simulink model "VehicleDynamics3D_controller"  (R2017a)
settings: Solver=ode45  StartTime=0.0  StopTime=stoptime  FixedStep=.001  MaxStep=maxStep  RelTol=relTol  AbsTol=absTol  EnableMultiTasking=on
PreLoadFcn:
  | VehicleDynamicsInitialization
model workspace: external: MATLAB File sm_suspension_templates_params.m (data not in the file)
values from neighbouring files (symbols this model uses):
  D = 0.1341    [Run_VehicleDynamics3D.m]
  Dt = 0.65979    [Run_VehicleDynamics3D.m]
  I = 0.55564    [Run_VehicleDynamics3D.m]
  It = 0.7671    [Run_VehicleDynamics3D.m]
  latv_setpoint = -12.28    [Run_VehicleDynamics3D.m]
  max_speed = 80    [Run_VehicleDynamics3D.m]
  P = 1.2095    [Run_VehicleDynamics3D.m]
  Pt = 2.1389    [Run_VehicleDynamics3D.m]
  ste_gain = 1    [Run_VehicleDynamics3D.m]
  steering_step = -30    [Run_VehicleDynamics3D.m]
  switch_speed_control = 3.28    [Run_VehicleDynamics3D.m]
  switch_steering = 100    [Run_VehicleDynamics3D.m]
  switch_steering_control = 3.58    [Run_VehicleDynamics3D.m]
  switch_throttle = 3.28    [Run_VehicleDynamics3D.m]
  thl_gain = 1    [Run_VehicleDynamics3D.m]
undefined symbols (not defined in the file or in its folder): dwb, Floor, followerCameraX, followerCameraZ, frontCameraX, frontCameraZ, isoCameraAimX, isoCameraX, isoCameraY, isoCameraZ, Load, maxSteeringDisplacement, minSteeringDisplacement, SetPaceSampleTime, wheel, wheelbase, X, Y, Z
libraries: sm_lib x199, sm_suspension_templates_lib x34, nesl_utility x20, simulink x8, fl_lib x7, Contact_Forces_Lib x4, aerolibanimutils x1
(part 1 of 7)
CloseFcn:
  | clear simlog_sm_suspension_templates
Description:
  | Independent Suspension System Templates
  | 
  | Copyright 2016-2017 The MathWorks, Inc.
settings Model: Creator=MathWorks  LastModifiedBy=regab
settings SolverCC: ZeroCrossAlgorithm=Adaptive
settings DataIOCC: SaveFormat=Array  SaveOutput=off  ReturnWorkspaceOutputs=on  ReturnWorkspaceOutputsName=FrameCopy_spidata
settings OptimizationCC: ExpressionDepthLimit=2147483647  LifeSpan=inf
settings DebuggingCC: UnderspecifiedInitializationDetection=Classic  MergeDetectMultiDrivingBlocksExec=none  MaskedZcDiagnostic=none  IgnoredZcDiagnostic=none  AllowSymbolicDim=off  StateNameClashWarn=warning  SFUnexpectedBacktrackingDiag=warning  SFNoUnconditionalDefaultTransitionDiag=warning  SFExecutionAtInitializationDiag=none
settings HardwareCC: ProdBitPerPointer=32  ProdBitPerSizeT=32  ProdBitPerPtrDiffT=32  ProdLargestAtomicFloat=None  ProdIntDivRoundTo=Undefined  ProdEndianess=Unspecified  ProdWordSize=32  ProdHWDeviceType=32-bit Generic
settings ModelReferenceCC: PropagateSignalLabelsOutOfModel=off
settings SFSimCC: SimBuildMode=sf_make
settings GRTTargetCC: TargetLangStandard=C89/C90 (ANSI)  GeneratePreprocessorConditionals=Disable all
settings ConfigComp: CovScope=ReferencedModels  CovIncludeTopModel=off  CovMetricSettings=dw  CovHtmlReporting=on  CovSaveCumulativeToWorkspaceVar=on  CovSaveSingleToWorkspaceVar=on  CovExternalEMLEnable=off  CovSFcnEnable=off
settings SimscapeCC: SimscapeLogSimulationStatistics=on  SimscapeLogLimitData=off  SimscapeLogDataHistory=10000
settings ConfigurationSet: Description=SimMechanics 2G
settings DiagnosticsConfigSet: SimMechanicsUnconnectedFramePorts=none  SimMechanicsRigidlyBoundBlock=none  SimMechanicsUnsatisfiedHighPriorityTargets=none
settings ExplorerConfigSet: InternalSimMechanicsExplorerSettings="<ExplorerConfiguration><canonicalview>default</canonicalview><AnimationSetting><BasePlaybackSpeed>1.0</BasePlaybackSpeed><PlaybackSpeedFactor>1.0</PlaybackSpeedFactor></AnimationSetting><TilePanel><TileInfo><Tiles Columns=\"2\" Count=\"3\" Rows=\"2\"><Column Left=\"2\" Weight=\"0.4529\"/><Column Left=\"381\" Weight=\"0.5471\"/><Column Left=\"837\"/><Row Top=\"2\" Weight=\"0.5729\"/><Row Top=\"598\" Weight=\"0.4271\"/><Row Top=\"1044\"/><Tile Height=\"2\" Width=\"1\" X=\"0\" Y=\"0\"/><Tile Height=\"1\" Width=\"1\" X=\"1\" Y=\"0\"/><Tile Height=\"1\" Width=\"1\" X=\"1\" Y=\"1\"/></Tiles></TileInfo><SceneInfo><SceneViewer><BGColor><R>0.60000002384185791</R><G>0.60000002384185791</G><B>0.60000002384185791</B></BGColor><Camera><DoPerspective>on</DoPerspective><Position><X>-1.1537063873740901e-15</X><Y>-7.5000000000000018</Y><Z>3.2999999999999994</Z></Position><Center><X>6.6613381477509392e-16</X><Y>1.1102230246251565e-16</Y><Z>0.29999999999999993</Z></Center><Up><X>-5.1501888403816389e-17</X><Y>-7.1161584930853499e-17</Y><Z>1</Z></Up><ViewLimDist>1</ViewLimDist><YLim>0.46630765815499858</YLim><XLim>0.16702210408262291</XLim></Camera></SceneViewer><SceneViewer><BGColor><R>0.60000002384185791</R><G>0.60000002384185791</G><B>0.60000002384185791</B></BGColor><Camera><DoPerspective>on</DoPerspective><Position><X>3.5000000000000018</X><Y>3.0999999999999996</Y><Z>1.8000000000000003</Z></Position><Center><X>4.9960036108132044e-16</X><Y>-0.75000000000000011</Y><Z>0.29999999999999988</Z></Center><Up><X>0</X><Y>0</Y><Z>1</Z></Up><ViewLimDist>1</ViewLimDist><YLim>0.46630765815499858</YLim><XLim>0.35509288448941123</XLim></Camera></SceneViewer><SceneViewer><BGColor><R>0.60000002384185791</R><G>0.60000002384185791</G><B>0.60000002384185791</B></BGColor><Camera><DoPerspective>on</DoPerspective><Position><X>1.036686212452563e-15</X><Y>1.7500000000000004</Y><Z>0.65000000000000002</Z></Position><Center><X>6.6613381477509392e-16</X><Y>1.1102230246251565e-16</Y><Z>0.29999999999999993</Z></Center><Up><X>-5.1501888403816389e-17</X><Y>-7.1161584930853499e-17</Y><Z>1</Z></Up><ViewLimDist>1</ViewLimDist><YLim>0.46630765815499858</YLim><XLim>0.47697831394801909</XLim></Camera></SceneViewer></SceneInfo></TilePanel><MechEditorPanel><Cameras><Camera><Id>Camera1</Id><Value><Name>Follower Camera</Name><NativeCamera><PositionTrackingFeature>Cameras.Follower_Camera_Transform.F</PositionTrackingFeature><CenterTrackingFeature>Cameras.Follower_Camera_Transform.B</CenterTrackingFeature><UpVectorTrackingFeature>Cameras.Follower_Camera_Transform.B</UpVectorTrackingFeature><CenterTrackingOrigin>on</CenterTrackingOrigin><UpVectorTrackingDirection>+Z</UpVectorTrackingDirection></NativeCamera></Value></Camera><Camera><Id>Camera2</Id><Value><Name>Isometric Camera</Name><NativeCamera><PositionTrackingFeature>Cameras.Isometric_Camera_Transform.F</PositionTrackingFeature><CenterTrackingFeature>Cameras.Isometric_Camera_Aim.F</CenterTrackingFeature><UpVectorTrackingFeature>Floor_And_Grid.World_Frame.W</UpVectorTrackingFeature><CenterTrackingOrigin>on</CenterTrackingOrigin><UpVectorTrackingDirection>+Z</UpVectorTrackingDirection></NativeCamera></Value></Camera><Camera><Id>Camera3</Id><Value><Name>Front Camera</Name><NativeCamera><PositionTrackingFeature>Cameras.Front_Camera_Transform.F</PositionTrackingFeature><CenterTrackingFeature>Cameras.Front_Camera_Transform.B</CenterTrackingFeature><UpVectorTrackingFeature>Cameras.Front_Camera_Transform.B</UpVectorTrackingFeature><CenterTrackingOrigin>on</CenterTrackingOrigin><UpVectorTrackingDirection>+Z</UpVectorTrackingDirection></NativeCamera></Value></Camera></Cameras><GfxPanelCameraMap><MapElement CameraMLId=\"Camera1\" GfxPanelIndex=\"0\"/><MapElement CameraMLId=\"Camera2\" GfxPanelIndex=\"1\"/><MapElement CameraMLId=\"Camera3\" GfxPanelIndex=\"2\"/></GfxPanelCameraMap><VideoCreator><PlaybackSpeedRatio>1.0</PlaybackSpeedRatio><FrameRate>30</FrameRate><VideoFormat>Motion JPEG AVI</VideoFormat><FrameSize>auto</FrameSize></VideoCreator></MechEditorPanel></ExplorerConfiguration>"

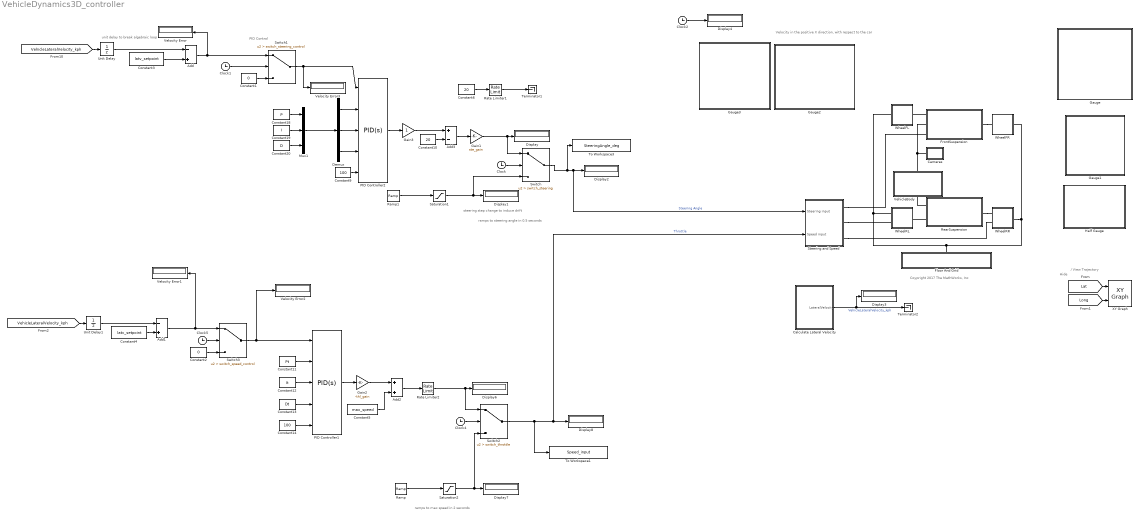
== system VehicleDynamics3D_controller ==
  note: Velocity in the positive X direction, with respect to the car
  note: Hide
  note: / View Trajectory
  note: Coypright 2017 The MathWorks, Inc
  note: ramps to max speed in 2 seconds
  note: unit delay to break algebraic loop
  note: steering step change to induce drift
  note: PID Control
  note: ramps to steering angle in 0.5 seconds
  Add : Sum  Inputs=-+
  Add1 : Sum  Inputs=-+
  Add2 : Sum
  Add3 : Sum  Inputs=+-
  Calculate Lateral Velocity : Subsystem
  Cameras : Subsystem
      mask Display: image('CameraPic.png');
  Clock{,1..2,4..5} (5 alike) : Clock
      Clock settings: Decimation=7
      Clock2 settings: Decimation=7
      Clock4 settings: Decimation=7
  Constant1 : Constant  Value=0
  Constant10 : Constant  Value=20
  Constant11 : Constant  Value=Pt  VectorParams1D=off
  Constant12 : Constant  Value=It
  Constant13 : Constant  Value=Dt
  Constant14 : Constant  Value=100
  Constant18 : Constant  Value=P
  Constant19 : Constant  Value=I
  Constant2 : Constant  Value=0
  Constant20 : Constant  Value=D
  Constant3 : Constant  Value=latv_setpoint
  Constant4 : Constant  Value=latv_setpoint
  Constant5 : Constant  Value=max_speed
  Constant6 : Constant  Value=20
  Constant9 : Constant  Value=100
  Demux : Demux  Outputs=3
  Display{,1..4,6..8} (8 alike) : Display
  Floor And Grid : Subsystem
      mask Display: image('Floor.png');
  FrontSuspension : Subsystem  VariantControl=DoubleWishbone
      mask Display:
      | image(imread(fullfile(matlabroot,...
      |     'toolbox','physmod','sm','smdemos',...
      |     'suspension_templates','images','sm_isuspension_dwishbone.png')));
  Gain1 : Gain  Gain=ste_gain
  Gain2 : Gain  Gain=-thl_gain
  Gain3 : Gain
  Gauge : Subsystem  DialogController=hmiCreateDDGDialog  IsWebBlock=on  mask(MWDashboardBlock){webBlockId=e0acaf17-1707-462e-bd3e-ad1907f2a35e, webBlockType=circulargauge, ShowInLibBrowser=on, ShowInitialText=on, HMISrcModelName=VehicleDynamics3D_controller}
      mask prompts: webBlockId "WebBlock Id"; webBlockType "WebBlock Type"; HMISrcModelName "Source Model"
      mask help: SimulinkHMI:dialogs:CircularGaugeDialogDesc
      mask Help: helpview([docroot '/mapfiles/simulink.map'], 'hmi_gauge')
      mask Display:
      | if strcmp(get_param(bdroot(gcb),'BlockDiagramType'), 'library')
      |     image([(matlabroot) '/toolbox/simulink/hmi/icons/CircularGauge.png']);
      | end
  Gauge1 : Subsystem  DialogController=hmiCreateDDGDialog  IsWebBlock=on  mask(MWDashboardBlock){webBlockId=a4d7a6c9-5cb1-4197-bb1e-6d17cd857777, webBlockType=circulargauge, ShowInLibBrowser=on, ShowInitialText=on, HMISrcModelName=VehicleDynamics3D_controller}
      mask prompts: webBlockId "WebBlock Id"; webBlockType "WebBlock Type"; HMISrcModelName "Source Model"
      mask help: SimulinkHMI:dialogs:CircularGaugeDialogDesc
      mask Help: helpview([docroot '/mapfiles/simulink.map'], 'hmi_gauge')
      mask Display:
      | if strcmp(get_param(bdroot(gcb),'BlockDiagramType'), 'library')
      |     image([(matlabroot) '/toolbox/simulink/hmi/icons/CircularGauge.png']);
      | end
  Gauge2 : Subsystem  DialogController=hmiCreateDDGDialog  IsWebBlock=on  mask(MWDashboardBlock){webBlockId=9138c855-01fc-4053-99a3-41b98eb70a74, webBlockType=circulargauge, ShowInLibBrowser=on, ShowInitialText=on, HMISrcModelName=VehicleDynamics3D_controller}
      mask prompts: webBlockId "WebBlock Id"; webBlockType "WebBlock Type"; HMISrcModelName "Source Model"
      mask help: SimulinkHMI:dialogs:CircularGaugeDialogDesc
      mask Help: helpview([docroot '/mapfiles/simulink.map'], 'hmi_gauge')
      mask Display:
      | if strcmp(get_param(bdroot(gcb),'BlockDiagramType'), 'library')
      |     image([(matlabroot) '/toolbox/simulink/hmi/icons/CircularGauge.png']);
      | end
  Gauge3 : Subsystem  DialogController=hmiCreateDDGDialog  IsWebBlock=on  mask(MWDashboardBlock){webBlockId=2bdbd2f3-79cc-4c0f-8469-e300a5d3b56d, webBlockType=circulargauge, ShowInLibBrowser=on, ShowInitialText=on, HMISrcModelName=VehicleDynamics3D_controller}
      mask prompts: webBlockId "WebBlock Id"; webBlockType "WebBlock Type"; HMISrcModelName "Source Model"
      mask help: SimulinkHMI:dialogs:CircularGaugeDialogDesc
      mask Help: helpview([docroot '/mapfiles/simulink.map'], 'hmi_gauge')
      mask Display:
      | if strcmp(get_param(bdroot(gcb),'BlockDiagramType'), 'library')
      |     image([(matlabroot) '/toolbox/simulink/hmi/icons/CircularGauge.png']);
      | end
  Half Gauge : Subsystem  DialogController=hmiCreateDDGDialog  IsWebBlock=on  mask(MWDashboardBlock){webBlockId=2bf35224-e477-42b1-a6f6-088c116ad7f4, webBlockType=semicirculargauge, ShowInLibBrowser=on, ShowInitialText=on, HMISrcModelName=VehicleDynamics3D_controller}
      mask prompts: webBlockId "WebBlock Id"; webBlockType "WebBlock Type"; HMISrcModelName "Source Model"
      mask help: SimulinkHMI:dialogs:SemicircularGaugeDialogDesc
      mask Help: helpview([docroot '/mapfiles/simulink.map'], 'hmi_half_gauge')
      mask Display:
      | if strcmp(get_param(bdroot(gcb),'BlockDiagramType'), 'library')
      |     image([(matlabroot) '/toolbox/simulink/hmi/icons/SemicircularGauge.png']);
      | end
  Mux1 : Mux  Inputs=3
  PID Controller1 : simulink/Continuous/PID Controller  Controller=PID  TimeDomain=Continuous-time  SampleTime=-1  IntegratorMethod=Forward Euler  FilterMethod=Forward Euler  Form=Parallel  UseFilter=on  ControllerParametersSource=external  P=.7*5  I=.2*4  D=1.2*3  N=100  InitialConditionSource=internal  InitialConditionForIntegrator=0  InitialConditionForFilter=0  ExternalReset=none  LimitOutput=on  UpperSaturationLimit=60  LowerSaturationLimit=-60  LinearizeAsGain=on  AntiWindupMode=none  Kb=4  TrackingMode=off  Kt=1  PParamMin=[]  PParamMax=[]  IParamMin=[]  IParamMax=[]  DParamMin=[]  DParamMax=[]  NParamMin=[]  NParamMax=[]  KbParamMin=[]  KbParamMax=[]  KtParamMin=[]  KtParamMax=[]  POutMin=[]  POutMax=[]  IOutMin=[]  IOutMax=[]  DOutMin=[]  DOutMax=[]  NOutMin=[]  NOutMax=[]  KbOutMin=[]  KbOutMax=[]  KtOutMin=[]  KtOutMax=[]  IntegratorOutMin=[]  IntegratorOutMax=[]  FilterOutMin=[]  FilterOutMax=[]  SumOutMin=[]  SumOutMax=[]  SumI1OutMin=[]  SumI1OutMax=[]  SumI2OutMin=[]  SumI2OutMax=[]  SumI3OutMin=[]  SumI3OutMax=[]  SumDOutMin=[]  SumDOutMax=[]  SaturationOutMin=[]  SaturationOutMax=[]  IntegratorContinuousStateAttributes=''  IntegratorStateMustResolveToSignalObject=off  IntegratorRTWStateStorageClass=Auto  FilterContinuousStateAttributes=''  FilterStateMustResolveToSignalObject=off  FilterRTWStateStorageClass=Auto  DifferentiatorICPrevScaledInput=0  DifferentiatorOutMin=[]  DifferentiatorOutMax=[]
  PID Controller2 : simulink/Continuous/PID Controller  Controller=PID  TimeDomain=Continuous-time  SampleTime=-1  IntegratorMethod=Forward Euler  FilterMethod=Forward Euler  Form=Parallel  UseFilter=on  ControllerParametersSource=external  P=.7*5  I=.2*4  D=1.2*3  N=100  InitialConditionSource=internal  InitialConditionForIntegrator=0  InitialConditionForFilter=0  ExternalReset=none  LimitOutput=on  UpperSaturationLimit=40  LowerSaturationLimit=-40  LinearizeAsGain=on  AntiWindupMode=none  Kb=1  TrackingMode=off  Kt=1  PParamMin=[]  PParamMax=[]  IParamMin=[]  IParamMax=[]  DParamMin=[]  DParamMax=[]  NParamMin=[]  NParamMax=[]  KbParamMin=[]  KbParamMax=[]  KtParamMin=[]  KtParamMax=[]  POutMin=[]  POutMax=[]  IOutMin=[]  IOutMax=[]  DOutMin=[]  DOutMax=[]  NOutMin=[]  NOutMax=[]  KbOutMin=[]  KbOutMax=[]  KtOutMin=[]  KtOutMax=[]  IntegratorOutMin=[]  IntegratorOutMax=[]  FilterOutMin=[]  FilterOutMax=[]  SumOutMin=[]  SumOutMax=[]  SumI1OutMin=[]  SumI1OutMax=[]  SumI2OutMin=[]  SumI2OutMax=[]  SumI3OutMin=[]  SumI3OutMax=[]  SumDOutMin=[]  SumDOutMax=[]  SaturationOutMin=[]  SaturationOutMax=[]  IntegratorContinuousStateAttributes=''  IntegratorStateMustResolveToSignalObject=off  IntegratorRTWStateStorageClass=Auto  FilterContinuousStateAttributes=''  FilterStateMustResolveToSignalObject=off  FilterRTWStateStorageClass=Auto  DifferentiatorICPrevScaledInput=0  DifferentiatorOutMin=[]  DifferentiatorOutMax=[]
  Ramp : simulink/Sources/Ramp  slope=max_speed/2  start=.75  X0=0
  Ramp1 : simulink/Sources/Ramp  slope=steering_step*2  start=steering_step_t  X0=0
  Rate Limiter1 : RateLimiter  RisingSlewLimit=500  FallingSlewLimit=-500  SampleTimeMode=inherited
  Rate Limiter2 : RateLimiter  RisingSlewLimit=50  FallingSlewLimit=-50  SampleTimeMode=inherited
  RearSuspension : Subsystem  VariantControl=DoubleWishbone
      mask Display:
      | image(imread(fullfile(matlabroot,...
      |     'toolbox','physmod','sm','smdemos',...
      |     'suspension_templates','images','sm_isuspension_dwishbone.png')));
  Saturation1 : Saturate  UpperLimit=abs(steering_step)  LowerLimit=-abs(steering_step)
  Saturation2 : Saturate  UpperLimit=max_speed  LowerLimit=0
  Steering and Speed : Subsystem
  Switch : Switch  Criteria=u2 > Threshold  Threshold=switch_steering
  Switch1 : Switch  Criteria=u2 > Threshold  Threshold=switch_steering_control  ZeroCross=off
  Switch2 : Switch  Criteria=u2 > Threshold  Threshold=switch_throttle
  Switch3 : Switch  Criteria=u2 > Threshold  Threshold=switch_speed_control  ZeroCross=off
  Terminator1 : Terminator
  Terminator2 : Terminator
  To Workspace1 : ToWorkspace  VariableName=Speed_input  SaveFormat=Timeseries  SampleTime=0.01
  To Workspace3 : ToWorkspace  VariableName=SteeringAngle_deg  SaveFormat=Timeseries  SampleTime=0.01
  Unit Delay : UnitDelay  SampleTime=-1
  Unit Delay1 : UnitDelay  SampleTime=-1
  VehicleBody : Subsystem
      mask Display: image('VehicleBodyPic.png');
  Velocity Error{,1..3} (4 alike) : Display
  WheelFL : Subsystem  mask(Wheel){Rti=wheel.tire.innerradius, Rto=wheel.tire.outerradius, Wt=wheel.tire.width, Rtr=wheel.tire.chamferradius, trho=wheel.tire.density, tclr=wheel.tire.color, Rhi=wheel.hub.radius, Rho=wheel.hub.outerradius, Ns=wheel.hub.numspokes, Ts=wheel.hub.spokethickness, Wh=wheel.hub.width, srho=wheel.hub.density, sclr=wheel.hub.color, Ls=wheel.shaft.length, Rs=wheel.shaft.radius, Rb=wheel.disc.radius, Tb=wheel.disc.thickness}
      mask prompts: Rti "Tire inner radius (cm):"; Rto "Tire outer radius (cm):"; Wt "Tire width (cm):"; Rtr "Chamfer/fillet radius (cm):"; trho "Density (kg/m^3):"; tclr "Color ([r  g b]):"; Rhi "Hub radius (cm):"; Rho "Outer radius of spokes (cm):"; Ns "Number of spokes:"; Ts "Thickness of spokes:"; Wh "Width of hub (cm):"; srho "Density (kg/m^3):"; sclr "Color ([r g b]):"; Ls "Shaft length (cm):"; Rs "Shaft radius (cm):"; Rb "Brake disc radius (cm):"; Tb "Brake disc thickness (cm):"
      mask help: This block models a wheel assembly. The port H corresponds to the center of the wheel hub. Port T corresponds to the bottom of the tire.
      mask init:
      | spk_angles = linspace(0,2*pi,Ns+1);
      | 
      | spokes_xsec = [];
      | r_indices = [];
      | wang = 20*pi/180;
      | for idx = 1:length(spk_angles)-1
      |     ang = spk_angles(idx);
      |     theta = linspace(ang-wang,ang+wang,20)';
      |     spokes_xsec = [spokes_xsec;
      |                    Rhi*cos(theta) Rhi*sin(theta)];
      |     theta = linspace(ang+wang, spk_angles(idx+1)-wang, 50)';
      |     len = length(spokes_xsec);
      |     r_indices = [r_indices len len+1];
      |     spokes_xsec = [spokes_xsec;
      |                    Rho*cos(theta) Rho*sin(theta)];
      | end
      | 
      | rim_xsec = [Rho -Wh/2; Rti -Wt/2; 
      |             Rti Wt/2; Rho Wh/2+Ts];
      | 
      | tire_xsec = [Rti -Wt/2; Rto -Wt/2; Rto Wt/2; Rti Wt/2];
      | tire_xsec = simmechanics.demohelpers.round_corners(tire_xsec,1:4,Rtr,10);
      mask Display:
      | image(imread(fullfile(matlabroot,...
      |     'toolbox','physmod','sm','smdemos',...
      |     'suspension_templates','images','sm_isuspension_wheel.png')));
      | 
      | port_label('LConn',1,'H');
      | port_label('RConn',1,'T');
  WheelFR : Subsystem  mask(Wheel){Rti=wheel.tire.innerradius, Rto=wheel.tire.outerradius, Wt=wheel.tire.width, Rtr=wheel.tire.chamferradius, trho=wheel.tire.density, tclr=wheel.tire.color, Rhi=wheel.hub.radius, Rho=wheel.hub.outerradius, Ns=wheel.hub.numspokes, Ts=wheel.hub.spokethickness, Wh=wheel.hub.width, srho=wheel.hub.density, sclr=wheel.hub.color, Ls=wheel.shaft.length, Rs=wheel.shaft.radius, Rb=wheel.disc.radius, Tb=wheel.disc.thickness}
      mask prompts: Rti "Tire inner radius (cm):"; Rto "Tire outer radius (cm):"; Wt "Tire width (cm):"; Rtr "Chamfer/fillet radius (cm):"; trho "Density (kg/m^3):"; tclr "Color ([r  g b]):"; Rhi "Hub radius (cm):"; Rho "Outer radius of spokes (cm):"; Ns "Number of spokes:"; Ts "Thickness of spokes:"; Wh "Width of hub (cm):"; srho "Density (kg/m^3):"; sclr "Color ([r g b]):"; Ls "Shaft length (cm):"; Rs "Shaft radius (cm):"; Rb "Brake disc radius (cm):"; Tb "Brake disc thickness (cm):"
      mask help: This block models a wheel assembly. The port H corresponds to the center of the wheel hub. Port T corresponds to the bottom of the tire.
      mask init: same as VehicleDynamics3D_controller/WheelFL
      mask Display:
      | image(imread(fullfile(matlabroot,...
      |     'toolbox','physmod','sm','smdemos',...
      |     'suspension_templates','images','sm_isuspension_wheel.png')));
      | 
      | port_label('LConn',1,'H');
      | port_label('RConn',1,'T');
  WheelRL : Subsystem  mask(Wheel){Rti=wheel.tire.innerradius, Rto=wheel.tire.outerradius, Wt=wheel.tire.width, Rtr=wheel.tire.chamferradius, trho=wheel.tire.density, tclr=wheel.tire.color, Rhi=wheel.hub.radius, Rho=wheel.hub.outerradius, Ns=wheel.hub.numspokes, Ts=wheel.hub.spokethickness, Wh=wheel.hub.width, srho=wheel.hub.density, sclr=wheel.hub.color, Ls=wheel.shaft.length, Rs=wheel.shaft.radius, Rb=wheel.disc.radius, Tb=wheel.disc.thickness}
      mask prompts: Rti "Tire inner radius (cm):"; Rto "Tire outer radius (cm):"; Wt "Tire width (cm):"; Rtr "Chamfer/fillet radius (cm):"; trho "Density (kg/m^3):"; tclr "Color ([r  g b]):"; Rhi "Hub radius (cm):"; Rho "Outer radius of spokes (cm):"; Ns "Number of spokes:"; Ts "Thickness of spokes:"; Wh "Width of hub (cm):"; srho "Density (kg/m^3):"; sclr "Color ([r g b]):"; Ls "Shaft length (cm):"; Rs "Shaft radius (cm):"; Rb "Brake disc radius (cm):"; Tb "Brake disc thickness (cm):"
      mask help: This block models a wheel assembly. The port H corresponds to the center of the wheel hub. Port T corresponds to the bottom of the tire.
      mask init: same as VehicleDynamics3D_controller/WheelFL
      mask Display:
      | image(imread(fullfile(matlabroot,...
      |     'toolbox','physmod','sm','smdemos',...
      |     'suspension_templates','images','sm_isuspension_wheel.png')));
      | 
      | port_label('LConn',1,'H');
      | port_label('RConn',1,'T');
  WheelRR : Subsystem  mask(Wheel){Rti=wheel.tire.innerradius, Rto=wheel.tire.outerradius, Wt=wheel.tire.width, Rtr=wheel.tire.chamferradius, trho=wheel.tire.density, tclr=wheel.tire.color, Rhi=wheel.hub.radius, Rho=wheel.hub.outerradius, Ns=wheel.hub.numspokes, Ts=wheel.hub.spokethickness, Wh=wheel.hub.width, srho=wheel.hub.density, sclr=wheel.hub.color, Ls=wheel.shaft.length, Rs=wheel.shaft.radius, Rb=wheel.disc.radius, Tb=wheel.disc.thickness}
      mask prompts: Rti "Tire inner radius (cm):"; Rto "Tire outer radius (cm):"; Wt "Tire width (cm):"; Rtr "Chamfer/fillet radius (cm):"; trho "Density (kg/m^3):"; tclr "Color ([r  g b]):"; Rhi "Hub radius (cm):"; Rho "Outer radius of spokes (cm):"; Ns "Number of spokes:"; Ts "Thickness of spokes:"; Wh "Width of hub (cm):"; srho "Density (kg/m^3):"; sclr "Color ([r g b]):"; Ls "Shaft length (cm):"; Rs "Shaft radius (cm):"; Rb "Brake disc radius (cm):"; Tb "Brake disc thickness (cm):"
      mask help: This block models a wheel assembly. The port H corresponds to the center of the wheel hub. Port T corresponds to the bottom of the tire.
      mask init: same as VehicleDynamics3D_controller/WheelFL
      mask Display:
      | image(imread(fullfile(matlabroot,...
      |     'toolbox','physmod','sm','smdemos',...
      |     'suspension_templates','images','sm_isuspension_wheel.png')));
      | 
      | port_label('LConn',1,'H');
      | port_label('RConn',1,'T');
  XY Graph : simulink/Sinks/XY Graph  xmin=lat_xmin  xmax=lat_xmax  ymin=lat_ymin  ymax=lat_ymax  st=0.5
  wires:
  [Lat] -> XY Graph/1
  [Long] -> XY Graph/2
  Calculate Lateral Velocity/1(LateralVelocity) -> Display3/1, Terminator2/1  "VehicleLateralVelocity_kph"
  Clock2/1 -> Display4/1
  Switch/1 -> To Workspace3/1, Steering and Speed/1(Steering input), Display2/1  "Steering Angle"
  Mux1/1 -> Demux/1
  Constant20/1 -> Mux1/3
  Constant14/1 -> PID Controller1/5
  Constant19/1 -> Mux1/2
  Demux/3 -> PID Controller2/4
  Constant12/1 -> PID Controller1/3
  Constant10/1 -> Add3/2
  Ramp/1 -> Saturation2/1
  Demux/1 -> PID Controller2/2
  Constant13/1 -> PID Controller1/4
  Add/1 -> Switch1/1, Velocity Error/1
  PID Controller2/1 -> Gain3/1
  Rate Limiter1/1 -> Terminator1/1
  Switch3/1 -> Velocity Error2/1, PID Controller1/1
  Clock/1 -> Switch/2
  Constant11/1 -> PID Controller1/2
  Rate Limiter2/1 -> Switch2/1, Display6/1
  [VehicleLateralVelocity_kph] -> Unit Delay/1
  Constant1/1 -> Switch1/3
  Gain1/1 -> Switch/1, Display/1
  Constant3/1 -> Add/2
  Gain3/1 -> Add3/1
  PID Controller1/1 -> Gain2/1
  Switch2/1 -> Steering and Speed/2(Speed input), Display8/1, To Workspace1/1  "Throttle"
  Switch1/1 -> PID Controller2/1, Velocity Error3/1
  Gain2/1 -> Add2/1
  Saturation2/1 -> Display7/1, Switch2/3
  Saturation1/1 -> Switch/3, Display1/1
  Constant6/1 -> Rate Limiter1/1
  [VehicleLateralVelocity_kph] -> Unit Delay1/1
  Clock4/1 -> Switch2/2
  Ramp1/1 -> Saturation1/1
  Constant5/1 -> Add2/2
  Demux/2 -> PID Controller2/3
  Add1/1 -> Velocity Error1/1, Switch3/1
  Constant4/1 -> Add1/2
  Clock1/1 -> Switch1/2
  Constant2/1 -> Switch3/3
  Constant9/1 -> PID Controller2/5
  Clock5/1 -> Switch3/2
  Add3/1 -> Gain1/1
  Add2/1 -> Rate Limiter2/1
  Unit Delay1/1 -> Add1/1
  Unit Delay/1 -> Add/1
  Constant18/1 -> Mux1/1
  connections:
  FrontSuspension/LConn1 -- WheelFL/LConn1
  FrontSuspension/RConn1 -- WheelFR/LConn1
  RearSuspension/RConn1 -- WheelRR/LConn1
  WheelRL/RConn1 -- WheelFL/RConn1 -- WheelRR/RConn1 -- WheelFR/RConn1 -- Floor And Grid/RConn1
  RearSuspension/LConn2 -- WheelRL/LConn1
  Cameras/LConn1 -- VehicleBody/LConn1 -- FrontSuspension/LConn2
  RearSuspension/LConn1 -- VehicleBody/RConn1
  Steering and Speed/RConn2 -- WheelRL/RConn2
  Steering and Speed/RConn3 -- WheelRR/LConn2
  Steering and Speed/RConn1 -- FrontSuspension/LConn3

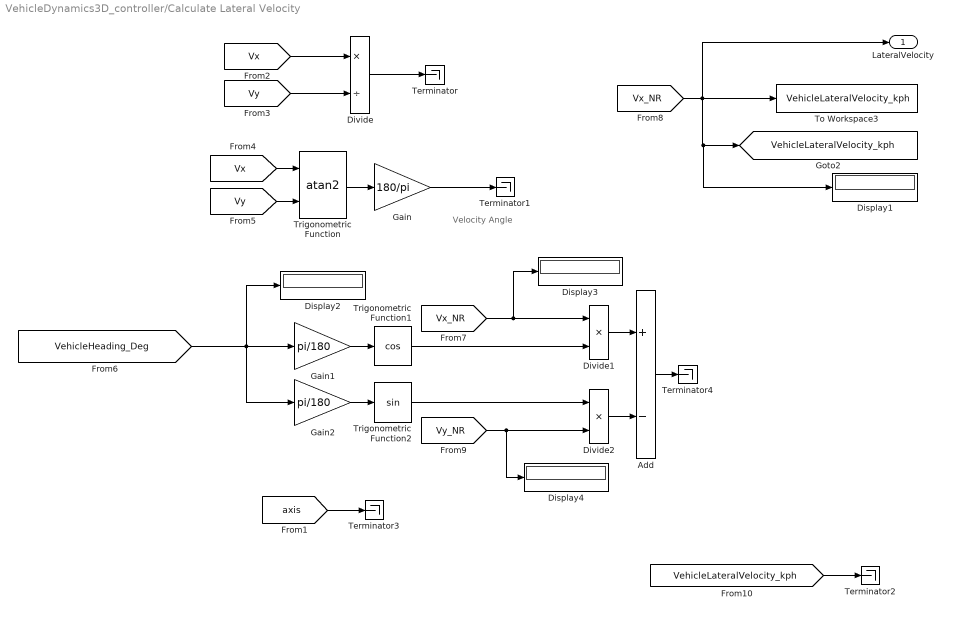
== system VehicleDynamics3D_controller/Calculate Lateral Velocity ==
  note: Velocity Angle
  Add : Sum  Inputs=+-
  Display{1..4} (4 alike) : Display
  Divide : Product  Inputs=*/
  Divide1 : Product  Inputs=**
  Divide2 : Product  Inputs=**
  Gain : Gain  Gain=180/pi
  Gain1 : Gain  Gain=pi/180
  Gain2 : Gain  Gain=pi/180
  Terminator{,1..4} (5 alike) : Terminator
  To Workspace3 : ToWorkspace  VariableName=VehicleLateralVelocity_kph  SaveFormat=Timeseries  SampleTime=0.01
  Trigonometric Function : Trigonometry  Operator=atan2
  Trigonometric Function1 : Trigonometry  Operator=cos
  Trigonometric Function2 : Trigonometry
  LateralVelocity : Outport
  tag scope: VehicleLateralVelocity_kph=global
  wires:
  [Vx_NR] -> Display3/1, Divide1/1
  Gain2/1 -> Trigonometric Function2/1
  [VehicleLateralVelocity_kph] -> Terminator2/1
  [Vy_NR] -> Display4/1, Divide2/2
  Divide/1 -> Terminator/1
  [Vy] -> Divide/2
  Trigonometric Function/1 -> Gain/1
  [Vy] -> Trigonometric Function/2
  Trigonometric Function1/1 -> Divide1/2
  Gain1/1 -> Trigonometric Function1/1
  Gain/1 -> Terminator1/1
  [Vx] -> Divide/1
  [Vx] -> Trigonometric Function/1
  Divide2/1 -> Add/2
  Trigonometric Function2/1 -> Divide2/1
  Divide1/1 -> Add/1
  [VehicleHeading_Deg] -> Display2/1, Gain2/1, Gain1/1
  [axis] -> Terminator3/1
  [Vx_NR] -> LateralVelocity/1, Display1/1, [VehicleLateralVelocity_kph], To Workspace3/1
  Add/1 -> Terminator4/1

== system VehicleDynamics3D_controller/Cameras ==
  Follower Camera Transform : sm_lib/Frames and Transforms/Rigid Transform  TranslationMethod=Cartesian  TranslationStandardOffset=0  TranslationLengthUnit=m  TranslationStandardAxis=+Z  TranslationCartesianOffset=[followerCameraX 0 followerCameraZ ]  TranslationROffset=0  TranslationROffsetUnits=m  TranslationZOffset=0  TranslationZOffsetUnits=m  TranslationThetaOffset=0  TranslationThetaOffsetUnits=deg  RotationMethod=None  RotationAngleUnits=deg  RotationStandardAxis=+Z  RotationAngle=0.0  RotationArbitraryAxis=[0 0 1]  FollAlignAxisA=+X  BaseAlignAxisA=+Y  FollAlignAxisB=+Y  BaseAlignAxisB=+Z  RotationSequenceAxes=FollowerAxes  RotationSequence=XYX  RotationSequenceAngles=[0 0 0]  RotationSequenceAnglesUnits=deg  RotationMatrix=[1 0 0; 0 1 0; 0 0 1]
  Front Camera Transform : sm_lib/Frames and Transforms/Rigid Transform  TranslationMethod=Cartesian  TranslationStandardOffset=0  TranslationLengthUnit=m  TranslationStandardAxis=+Z  TranslationCartesianOffset=[frontCameraX 0 frontCameraZ]  TranslationROffset=0  TranslationROffsetUnits=m  TranslationZOffset=0  TranslationZOffsetUnits=m  TranslationThetaOffset=0  TranslationThetaOffsetUnits=deg  RotationMethod=None  RotationAngleUnits=deg  RotationStandardAxis=+Z  RotationAngle=0.0  RotationArbitraryAxis=[0 0 1]  FollAlignAxisA=+X  BaseAlignAxisA=+Y  FollAlignAxisB=+Y  BaseAlignAxisB=+Z  RotationSequenceAxes=FollowerAxes  RotationSequence=XYX  RotationSequenceAngles=[0 0 0]  RotationSequenceAnglesUnits=deg  RotationMatrix=[1 0 0; 0 1 0; 0 0 1]
  Isometric Camera Transform : sm_lib/Frames and Transforms/Rigid Transform  TranslationMethod=Cartesian  TranslationStandardOffset=0  TranslationLengthUnit=m  TranslationStandardAxis=+Z  TranslationCartesianOffset=[isoCameraX isoCameraY isoCameraZ]  TranslationROffset=0  TranslationROffsetUnits=m  TranslationZOffset=0  TranslationZOffsetUnits=m  TranslationThetaOffset=0  TranslationThetaOffsetUnits=deg  RotationMethod=None  RotationAngleUnits=deg  RotationStandardAxis=+Z  RotationAngle=0.0  RotationArbitraryAxis=[0 0 1]  FollAlignAxisA=+X  BaseAlignAxisA=+Y  FollAlignAxisB=+Y  BaseAlignAxisB=+Z  RotationSequenceAxes=FollowerAxes  RotationSequence=XYX  RotationSequenceAngles=[0 0 0]  RotationSequenceAnglesUnits=deg  RotationMatrix=[1 0 0; 0 1 0; 0 0 1]
  Isometric Camera Aim : sm_lib/Frames and Transforms/Rigid Transform  TranslationMethod=Cartesian  TranslationStandardOffset=0  TranslationLengthUnit=m  TranslationStandardAxis=+Z  TranslationCartesianOffset=[isoCameraAimX 0 0]  TranslationROffset=0  TranslationROffsetUnits=m  TranslationZOffset=0  TranslationZOffsetUnits=m  TranslationThetaOffset=0  TranslationThetaOffsetUnits=deg  RotationMethod=None  RotationAngleUnits=deg  RotationStandardAxis=+Z  RotationAngle=0.0  RotationArbitraryAxis=[0 0 1]  FollAlignAxisA=+X  BaseAlignAxisA=+Y  FollAlignAxisB=+Y  BaseAlignAxisB=+Z  RotationSequenceAxes=FollowerAxes  RotationSequence=XYX  RotationSequenceAngles=[0 0 0]  RotationSequenceAnglesUnits=deg  RotationMatrix=[1 0 0; 0 1 0; 0 0 1]
  PS Integrator : fl_lib/Physical Signals/Linear Operators/PS Integrator  x0=0
      settings: SourceProductName=Simscape  SourceProductBaseCode=SS
  Revolute Joint : sm_lib/Joints/Revolute Joint  SenseConstraintForce=off  SenseConstraintForceX=off  SenseConstraintForceY=off  SenseConstraintForceZ=off  SenseConstraintTorque=off  SenseConstraintTorqueX=off  SenseConstraintTorqueY=off  SenseConstraintTorqueZ=off  SenseTotalForce=off  SenseTotalForceX=off  SenseTotalForceY=off  SenseTotalForceZ=off  SenseTotalTorque=off  SenseTotalTorqueX=off  SenseTotalTorqueY=off  SenseTotalTorqueZ=off  CompositeWrenchDir=FollowerOnBase  CompositeWrenchFrame=BaseFrame  EquilibriumPosition=0  EquilibriumPositionUnits=deg  SpringStiffness=IsoCameraStiffness  SpringStiffnessUnits=N*m/deg  DampingCoefficient=IsoCameraDamping  DampingCoefficientUnits=N*m/(deg/s)  TorqueActuationMode=ComputedTorque  MotionActuationMode=InputMotion  SensePosition=off  SenseVelocity=off  SenseAcceleration=off  SenseTorqueForce=off  PositionTargetSpecify=off  PositionTargetPriority=High  PositionTargetValue=0  PositionTargetValueUnits=deg  VelocityTargetSpecify=off  VelocityTargetPriority=High  VelocityTargetValue=0  VelocityTargetValueUnits=deg/s
  Solid : sm_lib/Body Elements/Solid  InertiaType=PointMass  Mass=1E-03  MassUnits=kg  CenterOfMass=[0 0 0]  CenterOfMassUnits=m  MomentsOfInertia=[1 1 1]  MomentsOfInertiaUnits=kg*m^2  ProductsOfInertia=[1 1 1]  ProductsOfInertiaUnits=kg*m^2  DensityBased=on  Density=1000  DensityUnits=kg/m^3  DoExposeReferenceFrame=on  SerializedFrames=<Frames/>  GraphicType=FromGeometry  MarkerShape=Sphere  MarkerSize=10  GraphicVisPropType=SimpleVisualProperties  GraphicDiffuseColor=[0.5 0.5 0.5]  GraphicSpecularColor=[0.5 0.5 0.5 1.0]  GraphicAmbientColor=[0.15 0.15 0.15 1.0]  GraphicEmissiveColor=[0.0 0.0 0.0 1.0]  GraphicShininess=75  GraphicOpacity=0  GeometryShape=Brick  RectangleSize=[1 1]  RectangleSizeUnits=m  BrickDimensions=[1 1 1]  BrickDimensionUnits=mm  CylinderRadius=1  CylinderRadiusUnits=m  CylinderLength=1  CylinderLengthUnits=m  SphereRadius=1  SphereRadiusUnits=m  EllipsoidRadii=[1 1 1]  EllipsoidRadiiUnits=m  ExtrusionCrossSection=[1 1; -1 1; -1 -1; 1 -1]  ExtrusionCrossSectionUnits=m  ExtrusionLength=1  ExtrusionLengthUnits=m  PolygonNumSides=3  PolygonOuterRadius=1  PolygonOuterRadiusUnits=m  ExtGeomFileType=STEP  ExtGeomFileUnits=m  RevolutionCrossSection=[1 1; 1 -1; 2 -1; 2 1]  RevolutionCrossSectionUnits=m  RevolutionExtent=Full  RevolutionAngle=180  RevolutionAngleUnits=deg
  Transform Sensor : sm_lib/Frames and Transforms/Transform Sensor  MeasurementFrame=Base  SenseAngle=off  SenseAxis=off  SenseAngle1=off  SenseAngle2=off  SenseAngle3=off  SenseQ=off  SenseR=off  SenseOmegaX=off  SenseOmegaY=off  SenseOmegaZ=on  SenseOmega1=off  SenseOmega2=off  SenseOmega3=off  SenseQDot=off  SenseRDot=off  SenseAlphaX=off  SenseAlphaY=off  SenseAlphaZ=off  SenseAlpha1=off  SenseAlpha2=off  SenseAlpha3=off  SenseQDDot=off  SenseRDDot=off  SenseX=off  SenseY=off  SenseZ=off  SenseRad=off  SenseAzim=off  SenseDist=off  SenseInc=off  SenseXDot=off  SenseYDot=off  SenseZDot=off  SenseRadDot=off  SenseAzimDot=off  SenseDistDot=off  SenseIncDot=off  SenseXDDot=off  SenseYDDot=off  SenseZDDot=off  SenseRadDDot=off  SenseAzimDDot=off  SenseDistDDot=off  SenseIncDDot=off
  " " : PMIOPort  Side=Left
  connections:
  Follower Camera Transform/LConn1 -- Isometric Camera Aim/LConn1 -- Revolute Joint/LConn1 -- Transform Sensor/LConn1 -- Front Camera Transform/LConn1 -- " "/RConn1
  Revolute Joint/RConn1 -- Solid/RConn1 -- Isometric Camera Transform/LConn1
  Transform Sensor/RConn2 -- PS Integrator/LConn1
  PS Integrator/RConn1 -- Revolute Joint/LConn2

== system VehicleDynamics3D_controller/Floor And Grid ==
  Floor : sm_lib/Body Elements/Solid  InertiaType=CalculateFromGeometry  Mass=1  MassUnits=kg  CenterOfMass=[0 0 0]  CenterOfMassUnits=m  MomentsOfInertia=[1 1 1]  MomentsOfInertiaUnits=kg*m^2  ProductsOfInertia=[0 0 0]  ProductsOfInertiaUnits=kg*m^2  DensityBased=on  Density=1000  DensityUnits=kg/(m^3)  DoExposeReferenceFrame=on  SerializedFrames=<Frames/>  GraphicType=FromGeometry  MarkerShape=Sphere  MarkerSize=10  MarkerSizeUnits=m  GraphicVisPropType=AdvancedVisualProperties  GraphicDiffuseColor=[0.6 0.6 0.6]  GraphicSpecularColor=[0.5 0.5 0.5 1.0]  GraphicAmbientColor=[0.15 0.15 0.15 1.0]  GraphicEmissiveColor=[0.0 0.0 0.0 1.0]  GraphicShininess=75  GraphicOpacity=1.0  GeometryShape=Brick  RectangleSize=[1 1]  RectangleSizeUnits=m  BrickDimensions=[Floor.l , Floor.w , Floor.h]  BrickDimensionUnits=m  CylinderRadius=1  CylinderRadiusUnits=m  CylinderLength=1  CylinderLengthUnits=m  SphereRadius=1  SphereRadiusUnits=m  EllipsoidRadii=[1 1 1]  EllipsoidRadiiUnits=m  ExtrusionCrossSection=[1 1; -1 1; -1 -1; 1 -1]  ExtrusionCrossSectionUnits=m  ExtrusionLength=1  ExtrusionLengthUnits=m  PolygonNumSides=3  PolygonOuterRadius=1  PolygonOuterRadiusUnits=m  ExtGeomFileType=STL  ExtGeomFileUnits=m  RevolutionCrossSection=[1 1; 1 -1; 2 -1; 2 1]  RevolutionCrossSectionUnits=m  RevolutionExtent=Full  RevolutionAngle=180  RevolutionAngleUnits=deg
  Grid : Subsystem
  Mechanism Configuration : sm_lib/Utilities/Mechanism Configuration  UniformGravity=Constant  GravityVector=[0 0 -9.80665]  GravityUnits=m/s^2  LinearizationDelta=0.001
  Solver Configuration : nesl_utility/Solver Configuration  PhysicalDomain=network_engine_domain  SubClassName=solver  LeftPortType=input  RightPortType=generic  Accelerate=off  Tones=[]  Harmonics=[]  SimulateNoise=off  Profile=off  UseLocalSampling=off  EnableSwitchedLinearOptims=on  FrequencyDomain=off  UseCCode=off  RelTol=0.001  AbsTol=1e-06  MinStep=1e-09  ToWorkspace=off  RevertToSquareIcSolve=off  NumHomotopyIterations=100  PhasorMode=off  PhasorModeNumHarmonics=1  OverrideAbsTol=off  DoDC=off  ResidualTolerance=1e-09  UseLocalSolver=off  LocalSolverChoice=NE_BACKWARD_EULER_ADVANCER  LocalSolverSampleTime=0.01  DoFixedCost=off  MaxNonlinIter=3  MaxModeIter=2  LinearAlgebra=Sparse  DelaysMemoryBudget=1024  AutomaticFiltering=on  FilteringTimeConstant=Filtering1Dto3DConnection
  World Frame : sm_lib/Frames and Transforms/World Frame
  R : PMIOPort  Side=Right
  connections:
  R/RConn1 -- Mechanism Configuration/RConn1 -- World Frame/RConn1 -- Solver Configuration/RConn1 -- Floor/RConn1 -- Grid/LConn1
